simulink model "dds_cwg_1k"  (R2016b)
(part 2 of 84)

  From43/1 -> pipeline7/1(d), pipeline4/1(d)
  pipeline7/1(q) -> snap_dds1/6(in_sync)
  pipeline4/1(q) -> snap_dds1/8(trig)
  pipeline5/1(q) -> snap_dds1/7(we)
  bus_expand5/1(msb_out8) -> snap_dds/1(in_p0_d0)
  bus_expand5/2(out7) -> snap_dds/2(in_p0_d1)
  bus_expand5/3(out6) -> snap_dds/3(in_p0_d2)
  bus_expand5/4(out5) -> snap_dds/4(in_p0_d3)
  bus_expand5/5(out4) -> snap_dds1/1(in_p0_d0)
  bus_expand5/6(out3) -> snap_dds1/2(in_p0_d1)
  bus_expand5/7(out2) -> snap_dds1/3(in_p0_d2)
  bus_expand5/8(lsb_out1) -> snap_dds1/4(in_p0_d3)
  Gateway Out34/1 -> To Workspace34/1
  Gateway Out35/1 -> To Workspace35/1
  Constant17/1 -> White Gaussian Noise/1
  Constant19/1 -> White Gaussian Noise/2
  White Gaussian Noise/1 -> Reinterpret/1
  Gateway Out36/1 -> To Workspace36/1
  Reinterpret/1 -> Slice/1
  gap_offset/1(in_offset) -> AddSub2/1, Mux/2
  Constant30/1 -> gap_sel/1(sim_1)
  gap_sel/1(in_sel) -> Mux/1
  Mux/1 -> Register/1
  Register/1 -> AddSub3/1, Gateway Out38/1
  Gateway Out37/1 -> To Workspace37/1
  Gateway Out38/1 -> To Workspace38/1
  Gateway Out39/1 -> To Workspace39/1
  Reinterpret1/1 -> Slice1/1
  White Gaussian Noise/2 -> Reinterpret1/1
  [pkt_len] -> Relational2/2
  Constant32/1 -> pkt_len_sel/1(sim_1)
  pkt_len_sel/1(in_sel) -> Mux1/1
  Constant33/1 -> pkt_len/1(sim_1)
  pkt_len/1(in_len) -> AddSub1/1, Mux1/2
  Gateway Out40/1 -> To Workspace40/1
  Mux1/1 -> Gateway Out40/1, [pkt_len]
  AddSub1/1 -> Mux1/3
  Slice1/1 -> AddSub1/2
  Delay1/1 -> edge_detect2/1(in)
  Slice/1 -> AddSub2/2
  AddSub2/1 -> Gateway Out36/1, Mux/3
  cwg_cos/2(data_out) -> [osc_cos_ddc0]
  cwg_sin/2(data_out) -> [osc_sin_ddc0]
  Slice2/1 -> nb_pfb/5(fft_shift)
  Constant9/1 -> freq_cwg_input/1(sim_1)
  Constant34/1 -> freq_cwg_osc/1(sim_1)
  Gateway Out41/1 -> To Workspace41/1
  cwg2/2(data_out) -> [cwg80]
  cwg2/3(dv_out) -> Gateway Out31/1, [ddc_dv_in]
